simulink model "Topo_02_pcm"  (R2013a)
settings: Solver=ode45  StartTime=0.0  StopTime=10.0  RelTol=1e-6
undefined symbols (not defined in the file): magnitude
(part 2 of 2)

== matlab function Topo_02_pcm/Subsystem1/Subsystem/ACPO_KL/Subsystem/R3/MATLAB Function1 ==
  data: x input; y input; theta input; xr output; yr output
function [xr,yr]=Rot_theta(x,y,theta)
xr=[cos(theta) -sin(theta)]*[x y]';
yr=[sin(theta) cos(theta)]*[x y]';
end

== matlab function Topo_02_pcm/Subsystem1/Subsystem/ACPO_KL/Subsystem/R2/MATLAB Function1 ==
  data: x input; y input; theta input; xr output; yr output
function [xr,yr]=Rot_theta(x,y,theta)
xr=[cos(theta) -sin(theta)]*[x y]';
yr=[sin(theta) cos(theta)]*[x y]';
end

== matlab function Topo_02_pcm/Subsystem1/Subsystem/ACPO_KL/Subsystem/R1/MATLAB Function1 ==
  data: x input; y input; theta input; xr output; yr output
function [xr,yr]=Rot_theta(x,y,theta)
xr=[cos(theta) -sin(theta)]*[x y]';
yr=[sin(theta) cos(theta)]*[x y]';
end

== matlab function Topo_02_pcm/Subsystem1/Subsystem/ACPO_KR/Subsystem/R3/MATLAB Function1 ==
  data: x input; y input; theta input; xr output; yr output
function [xr,yr]=Rot_theta(x,y,theta)
xr=[cos(theta) -sin(theta)]*[x y]';
yr=[sin(theta) cos(theta)]*[x y]';
end

== matlab function Topo_02_pcm/Subsystem1/MATLAB Function1 ==
  data: phi input; pcm output
function pcm=pcm(phi)
g=phi.*180./pi;
for i=1:length(g)
    if g(i)<0 
        g(i)=g(i)+360;
    end
end
pcm=g.*100./(360);

== matlab function Topo_02_pcm/Subsystem1/MATLAB Function2 ==
  data: phi input; pcm output
function pcm=pcm(phi)
g=phi.*180./pi;
for i=1:length(g)
    if g(i)<0 
        g(i)=g(i)+360;
    end
end
pcm=g.*100./(360);

== matlab function Topo_02_pcm/Subsystem1/MATLAB Function3 ==
  data: phi input; pcm output
function pcm=pcm(phi)
g=phi.*180./pi;
for i=1:length(g)
    if g(i)<0 
        g(i)=g(i)+360;
    end
end
pcm=g.*100./(360);
